simulink model "Question2_Not Working Properly Yet"  (R2016b)
settings: Solver=VariableStepAuto  StartTime=0.0  StopTime=10.0  RelTol=1e-3
settings Model: Creator=MUHAMMED  LastModifiedBy=MUHAMMED

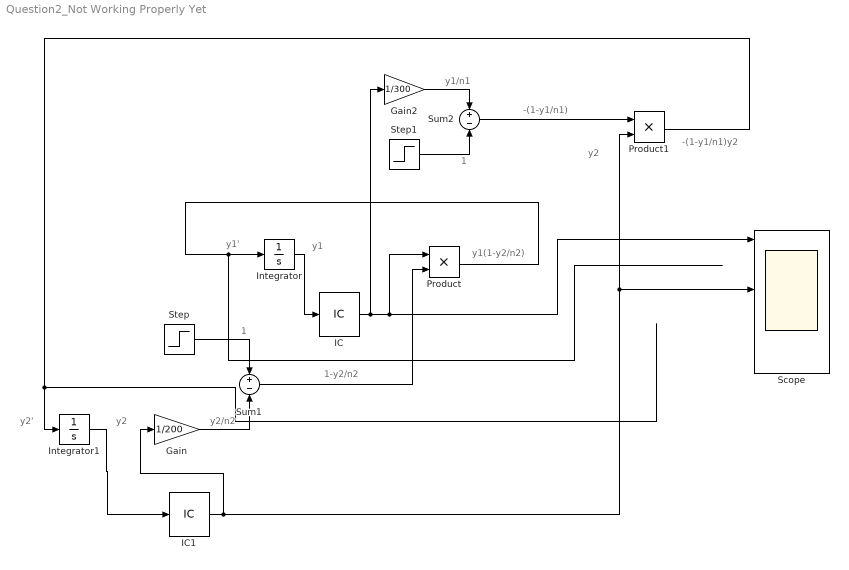
== system Question2_Not Working Properly Yet ==
  note: -(1-y1/n1)y2
  note: -(1-y1/n1)
  note: y1/n1
  note: 1
  note: y2
  note: y1(1-y2/n2)
  note: 1-y2/n2
  note: 1
  note: y1
  note: y1'
  note: y2'
  note: y2/n2
  note: y2
  Gain : Gain  Gain=1/200
  Gain2 : Gain  Gain=1/300
  IC : InitialCondition  Value=400
  IC1 : InitialCondition  Value=100
  Integrator : Integrator
  Integrator1 : Integrator
  Product : Product
  Product1 : Product
  Scope : Scope  NumInputPorts=6
  Step : Step  SampleTime=0
  Step1 : Step  SampleTime=0
  Sum1 : Sum  Inputs=+-
  Sum2 : Sum  Inputs=+-
  wires:
  Integrator1/1 -> IC1/1
  Gain/1 -> Sum1/2
  Step/1 -> Sum1/1
  Sum1/1 -> Product/2
  Integrator/1 -> IC/1
  Product/1 -> Integrator/1
  Gain2/1 -> Sum2/1
  Step1/1 -> Sum2/2
  Sum2/1 -> Product1/1
  Product1/1 -> Integrator1/1
  IC/1 -> Gain2/1, Product/1, Scope/1
  IC1/1 -> Scope/3, Product1/2, Gain/1
